simulink model "Sim_exercise4"  (R2015b)
settings: Solver=ode45  SolverMode=SingleTasking  StartTime=0.0  StopTime=10  RelTol=1e-3
values from neighbouring files (symbols this model uses):
  Amplitude = 2    [Exercise_3.m]
  dm = 3.8E-6    (= 3.8e-06)    [Exercise_1.m]    (also in Exercise_3.m)
  Freq = 2    [Exercise_3.m]
  Jeq = Jm + (J1+J2)/(n^2)    (= 2.186e-06)    [Exercise_1.m]    (also in Exercise_3.m)
  Kemf = 137*2*pi/60    (= 14.3466064514)    [Exercise_1.m]    (also in Exercise_3.m = 0.0697028947848)
  Km = 69.7E-3    (= 0.0697)    [Exercise_1.m]    (also in Exercise_3.m)
  n = 5    [Exercise_1.m]    (also in Exercise_3.m)
  R = 112    [Exercise_1.m]    (also in Exercise_3.m)
  Sine_wave = 1    [Exercise_3.m]
  voltage = 1    [Exercise_3.m]
undefined symbols (not defined in the file or in its folder): Ts
libraries: simulink x2
settings Model: Creator=sofianh  LastModifiedBy=sofianh
settings DataIOCC: SaveFormat=Array
settings OptimizationCC: BlockReduction=off  BooleanDataType=off
settings DebuggingCC: SaveWithParameterizedLinksMsg=none  UnderspecifiedInitializationDetection=Classic  MergeDetectMultiDrivingBlocksExec=none  SignalResolutionControl=TryResolveAllWithWarning
settings HardwareCC: ProdBitPerPointer=32  ProdLargestAtomicFloat=None  ProdIntDivRoundTo=Undefined  ProdEndianess=Unspecified  ProdWordSize=32  ProdHWDeviceType=32-bit Generic  TargetUnknown=on
settings GRTTargetCC: GeneratePreprocessorConditionals=Disable all
settings ConfigComp: CovModelRefEnable=Off  CovSFcnEnable=off

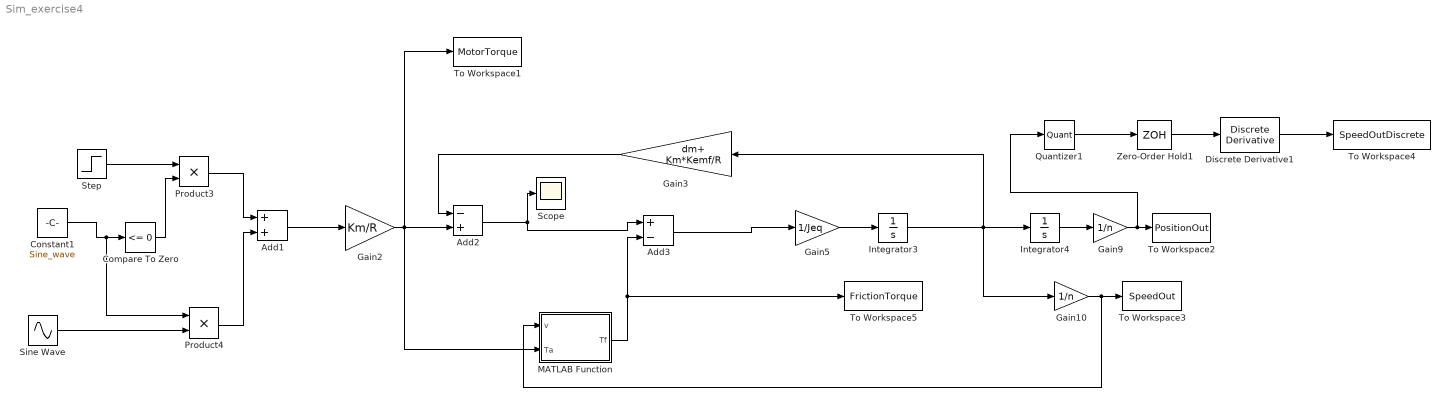
== system Sim_exercise4 ==
  Add1 : Sum
  Add2 : Sum  Inputs=-+
  Add3 : Sum  Inputs=+-
  Compare To Zero : simulink/Logic and Bit Operations/Compare To Zero  relop=<=  OutDataTypeStr=boolean
  Constant1 : Constant  Value=Sine_wave
  Discrete Derivative1 : simulink/Discrete/Discrete Derivative  gainval=1.0  ICPrevScaledInput=0.0  InputProcessing=Inherited  OutMin=[]  OutMax=[]  OutDataType=fixdt(1, 16)  OutScaling=2^-10  DoSatur=off
  Gain10 : Gain  Gain=1/n
  Gain2 : Gain  Gain=Km/R
  Gain3 : Gain  Gain=dm+ Km*Kemf/R
  Gain5 : Gain  Gain=1/Jeq
  Gain9 : Gain  Gain=1/n
  Integrator3 : Integrator
  Integrator4 : Integrator
  MATLAB Function : MATLAB Function  TreatAsAtomicUnit=on
  Product3 : Product
  Product4 : Product
  Quantizer1 : Quantizer  QuantizationInterval=Pulses  LinearizeAsGain=off  SampleTime=Ts
  Scope : Scope
  Sine Wave : Sin  Amplitude=Amplitude  Frequency=Freq  SampleTime=0
  Step : Step  Time=0  After=voltage  SampleTime=0
  To Workspace1 : ToWorkspace  VariableName=MotorTorque  SaveFormat=Structure With Time  SampleTime=-1
  To Workspace2 : ToWorkspace  VariableName=PositionOut  SaveFormat=Structure With Time  SampleTime=-1
  To Workspace3 : ToWorkspace  VariableName=SpeedOut  SaveFormat=Structure With Time  SampleTime=-1
  To Workspace4 : ToWorkspace  VariableName=SpeedOutDiscrete  SaveFormat=Structure With Time  SampleTime=-1
  To Workspace5 : ToWorkspace  VariableName=FrictionTorque  SaveFormat=Structure With Time  SampleTime=-1
  Zero-Order Hold1 : ZeroOrderHold  SampleTime=Ts
  wires:
  Integrator3/1 -> Integrator4/1, Gain10/1, Gain3/1
  Quantizer1/1 -> Zero-Order Hold1/1
  Zero-Order Hold1/1 -> Discrete Derivative1/1
  Discrete Derivative1/1 -> To Workspace4/1
  Gain2/1 -> MATLAB Function/2(Ta), To Workspace1/1, Add2/2
  Gain3/1 -> Add2/1
  Gain5/1 -> Integrator3/1
  Integrator4/1 -> Gain9/1
  Gain9/1 -> Quantizer1/1, To Workspace2/1
  Gain10/1 -> MATLAB Function/1(v), To Workspace3/1
  Step/1 -> Product3/1
  Constant1/1 -> Product4/1, Compare To Zero/1
  Sine Wave/1 -> Product4/2
  Product3/1 -> Add1/1
  Product4/1 -> Add1/2
  Compare To Zero/1 -> Product3/2
  Add1/1 -> Gain2/1
  Add3/1 -> Gain5/1
  Add2/1 -> Add3/1, Scope/1
  MATLAB Function/1(Tf) -> Add3/2, To Workspace5/1

== matlab function Sim_exercise4/MATLAB Function ==
  data: v input; Tf output; Ta input
function Tf = fcn(v,Ta)
Tc = 1e-3;
dv = 1e-1;
if abs(v) < dv
    if abs(Ta) > Tc
        Tf = Tc*sign(Ta);
    else
        Tf = Ta;
    end
else
    Tf = Tc*sign(v);
end
